simulink model "qrotor_dynamics"  (R2022a)
settings: Solver=VariableStepAuto  StartTime=0.0  StopTime=5  RelTol=1e-9
settings Model: Creator=carlossilvestre  LastModifiedBy=FLKU
settings SolverCC: AlgebraicLoopSolver=TrustRegion
settings DebuggingCC: UnconnectedInputMsg=warning  UnconnectedOutputMsg=warning  UnconnectedLineMsg=warning  SFMachineParentedDataDiag=warning

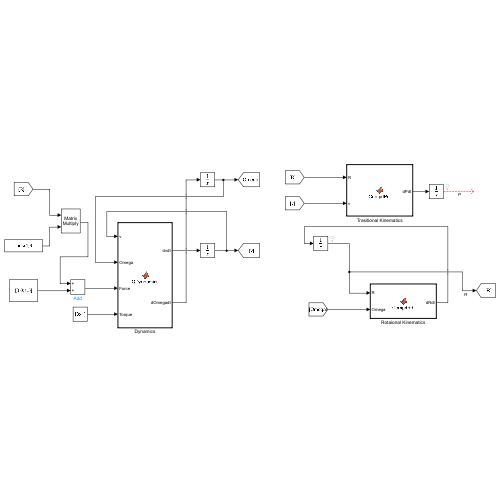
[thumbnail: Simulink's stored preview of the top-level diagram]
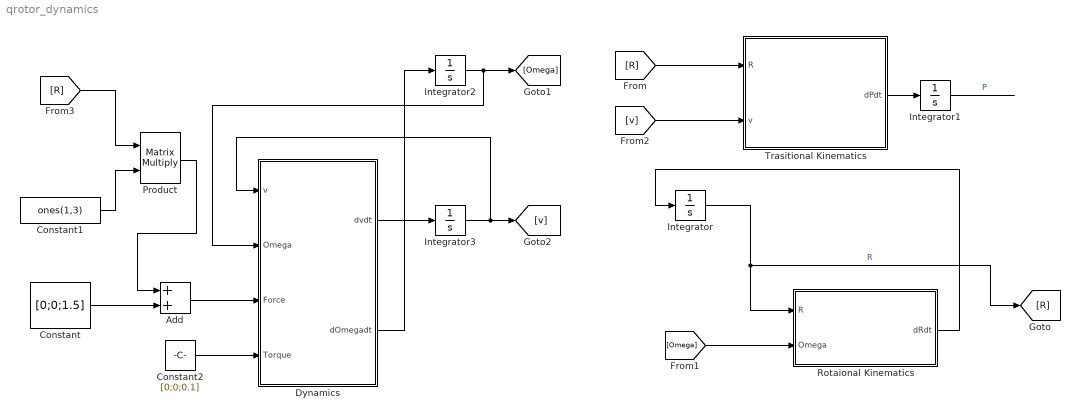
== system qrotor_dynamics ==
  Add : Sum
  Constant : Constant  Value=[0;0;1.5]
  Constant1 : Constant  Value=ones(1,3)
  Constant2 : Constant  Value=[0;0;0.1]
  Dynamics : MATLAB Function  TreatAsAtomicUnit=on
  Integrator : Integrator  InitialCondition=eye(3)
  Integrator1 : Integrator  InitialCondition=[0,0,0]
  Integrator2 : Integrator  InitialCondition=[0,0,0]  ContinuousStateAttributes='omega'
  Integrator3 : Integrator  InitialCondition=[0,0,0]  ContinuousStateAttributes='velocity'
  Product : Product  Multiplication=Matrix(*)
  Rotaional Kinematics : MATLAB Function  TreatAsAtomicUnit=on
  Trasitional Kinematics : MATLAB Function  TreatAsAtomicUnit=on
  wires:
  Dynamics/1(dvdt) -> Integrator3/1
  Integrator2/1 -> [Omega], Dynamics/2(Omega)
  Rotaional Kinematics/1(dRdt) -> Integrator/1
  Dynamics/2(dOmegadt) -> Integrator2/1
  [R] -> Trasitional Kinematics/1(R)
  Trasitional Kinematics/1(dPdt) -> Integrator1/1
  [Omega] -> Rotaional Kinematics/2(Omega)
  [v] -> Trasitional Kinematics/2(v)
  Integrator/1 -> Rotaional Kinematics/1(R), [R]  "R"
  Integrator3/1 -> [v], Dynamics/1(v)
  Product/1 -> Add/1
  Constant/1 -> Add/2
  Add/1 -> Dynamics/3(Force)
  Constant2/1 -> Dynamics/4(Torque)
  [R] -> Product/1
  Constant1/1 -> Product/2
  Integrator1/1 -> ?  "P"

== matlab function qrotor_dynamics/Trasitional Kinematics ==
  data: R input; dPdt output; v input
function dPdt = CompdPdt(R,v)
dPdt=R*v;
end

== matlab function qrotor_dynamics/Rotaional Kinematics ==
  data: R input; dRdt output; Omega input
function dRdt = CompdRdt(R,Omega)
dRdt=R*skew(Omega);
end

== matlab function qrotor_dynamics/Dynamics ==
  data: v input; Omega input; Force input; dvdt output; Torque input; dOmegadt output
function [dvdt,dOmegadt] = QDyanamics(v,Omega,Force,Torque)
m=0.1;
I=eye(3)*0.1;
dvdt=-skew(Omega)*v+1/m*Force;
dOmegadt=-I^-1*skew(Omega)*I*Omega+I^-1*Torque;
end
